simulink model "QUESTION1"  (R2020a)
settings: Solver=VariableStepAuto  StartTime=0.0  StopTime=10.0  RelTol=1e-3
model workspace (MAT data in the model file):
  K = Simulink.Parameter
  K.Value = 2000
  K.DataType = 'auto'
  K.Dimensions = [1 1]
  K1 = Simulink.Parameter
  K1.Value = 50
  K1.DataType = 'auto'
  K1.Dimensions = [1 1]
  M2 = Simulink.Parameter
  M2.Value = 20
  M2.DataType = 'auto'
  M2.Dimensions = [1 1]
  b = Simulink.Parameter
  b.Value = 50
  b.DataType = 'auto'
  b.Dimensions = [1 1]
settings Model: OrderedModelArguments=off  Creator=anjal  LastModifiedBy=anjal

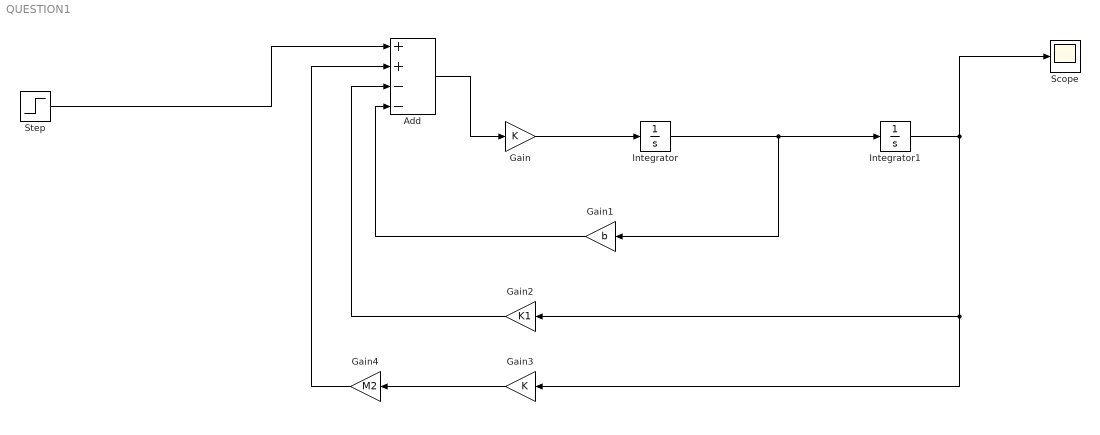
== system QUESTION1 ==
  Add : Sum  Inputs=++--
  Gain : Gain  Gain=K
  Gain1 : Gain  Gain=b
  Gain2 : Gain  Gain=K1
  Gain3 : Gain  Gain=K
  Gain4 : Gain  Gain=M2
  Integrator : Integrator  InitialCondition=100
  Integrator1 : Integrator  InitialCondition=50
  Scope : Scope
  Step : Step  After=10  SampleTime=0
  wires:
  Gain/1 -> Integrator/1
  Gain1/1 -> Add/4
  Add/1 -> Gain/1
  Step/1 -> Add/1
  Integrator1/1 -> Gain3/1, Gain2/1, Scope/1
  Gain3/1 -> Gain4/1
  Gain2/1 -> Add/3
  Gain4/1 -> Add/2
  Integrator/1 -> Gain1/1, Integrator1/1
